simulink model "glucosereg"  (Simulink 6.6)
settings: Solver=ode45  StartTime=0.0  StopTime=6000  MaxStep=10  RelTol=1e-19
settings Model: Creator=mxkana  LastModifiedBy=mxkana
settings DataIOCC: MaxDataPoints=10000000  SaveOutput=off  SaveTime=off  SignalLoggingName=sigsOut
settings DebuggingCC: SignalResolutionControl=TryResolveAllWithWarning  SolverPrmCheckMsg=none  MultiTaskDSMMsg=warning  MultiTaskCondExecSysMsg=none  StrictBusMsg=None
settings HardwareCC: TargetUnknown=on
settings RTWCC: IncludeERTFirstTime=on
settings GRTTargetCC: ModelReferenceCompliant=off  MatFileLogging=off

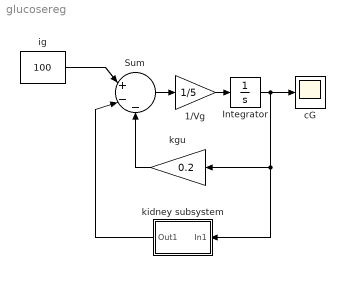
== system glucosereg ==
  1/Vg : Gain  Gain=1/5  SaturateOnIntegerOverflow=on
  Integrator : Integrator  InitialCondition=600
  Sum : Sum  Inputs=|+--  SaturateOnIntegerOverflow=on
  cG : Scope
      settings: TimeRange=15000  YMin=0  YMax=0.001
  ig : Constant  Value=100
  kgu : Gain  Orientation=left  Gain=0.2  SaturateOnIntegerOverflow=on
  kidney subsystem : Subsystem  Orientation=left
  wires:
  1/Vg/1 -> Integrator/1
  Integrator/1 -> cG/1, kgu/1, kidney subsystem/1(In1)
  Sum/1 -> 1/Vg/1
  kidney subsystem/1(Out1) -> Sum/2
  kgu/1 -> Sum/3
  ig/1 -> Sum/1

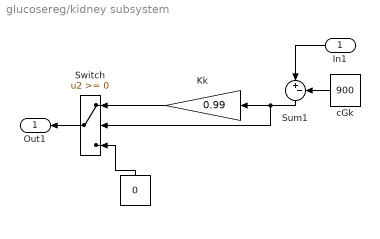
== system glucosereg/kidney subsystem ==
  In1 : Inport  Orientation=left
  " " : Constant  Orientation=up  Value=0
  Kk : Gain  Orientation=left  Gain=0.99  SaturateOnIntegerOverflow=on
  Sum1 : Sum  Orientation=down  Inputs=|+-  SaturateOnIntegerOverflow=on
  Switch : Switch  Orientation=left  SaturateOnIntegerOverflow=on
  cGk : Constant  Orientation=left  Value=900
  Out1 : Outport  Orientation=left
  wires:
  Sum1/1 -> Kk/1, Switch/2
  Switch/1 -> Out1/1
  " "/1 -> Switch/3
  Kk/1 -> Switch/1
  In1/1 -> Sum1/1
  cGk/1 -> Sum1/2
